simulink model "crearhuerto_Harness11"  (R2020b)
settings: Solver=VariableStepAuto  StartTime=0.0  StopTime=10.0  RelTol=1e-3
settings Model: Creator=Jose  LastModifiedBy=Jose

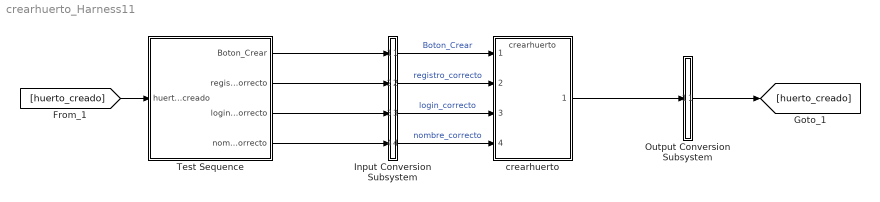
== system crearhuerto_Harness11 ==
  Input Conversion Subsystem : Subsystem  Tag=__SLT_ICS__  Description=|
      | Signal spec.
      | and routing
      settings: AttributesFormatString=%<Description>
  Output Conversion Subsystem : Subsystem  Tag=__SLT_OCS__  Description=|
      | Signal spec.
      | and routing
      settings: AttributesFormatString=%<Description>
  Test Sequence : Test Sequence  TreatAsAtomicUnit=on
  crearhuerto : ModelReference  ModelNameDialog=crearhuerto  SimulationMode=Normal  ModelReferenceVersion=1.12
  wires:
  Test Sequence/1(Boton_Crear) -> Input Conversion Subsystem/1(Inport_1)
  Test Sequence/2(registro_correcto) -> Input Conversion Subsystem/2(Inport_2)
  Test Sequence/3(login_correcto) -> Input Conversion Subsystem/3(Inport_3)
  Test Sequence/4(nombre_correcto) -> Input Conversion Subsystem/4(Inport_4)
  [huerto_creado] -> Test Sequence/1(huerto_creado)
  Output Conversion Subsystem/1(Outport_1) -> [huerto_creado]
  Input Conversion Subsystem/1(Outport_1) -> crearhuerto/1  "Boton_Crear"
  Input Conversion Subsystem/2(Outport_2) -> crearhuerto/2  "registro_correcto"
  Input Conversion Subsystem/3(Outport_3) -> crearhuerto/3  "login_correcto"
  Input Conversion Subsystem/4(Outport_4) -> crearhuerto/4  "nombre_correcto"
  crearhuerto/1 -> Output Conversion Subsystem/1(Inport_1)

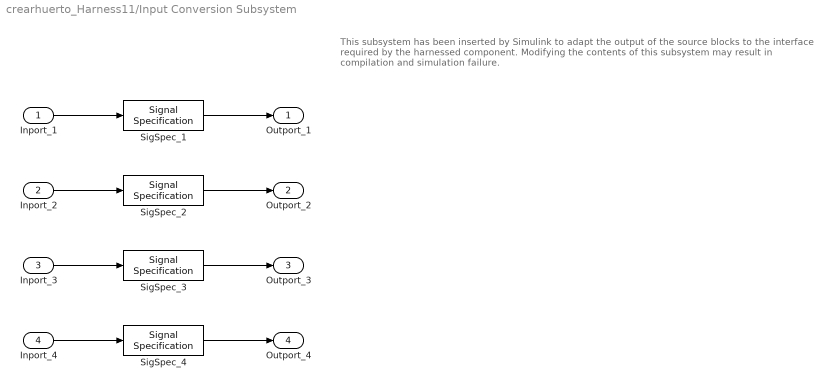
== system crearhuerto_Harness11/Input Conversion Subsystem ==
  note: This subsystem has been inserted by Simulink to adapt the output of the source blocks to the interface required by the harnessed component.
      |  Modifying the contents of this subsystem may result in compilation and simulation failure.
  Inport_1 : Inport
  Inport_2 : Inport  Port=2
  Inport_3 : Inport  Port=3
  Inport_4 : Inport  Port=4
  SigSpec_{1..4} (4 alike) : SignalSpecification  OutDataTypeStr=boolean  Dimensions=[1]  SampleTime=[-1, 0]
  Outport_1 : Outport
  Outport_2 : Outport  Port=2
  Outport_3 : Outport  Port=3
  Outport_4 : Outport  Port=4
  wires:
  SigSpec_1/1 -> Outport_1/1
  Inport_1/1 -> SigSpec_1/1
  SigSpec_2/1 -> Outport_2/1
  Inport_2/1 -> SigSpec_2/1
  SigSpec_3/1 -> Outport_3/1
  Inport_3/1 -> SigSpec_3/1
  SigSpec_4/1 -> Outport_4/1
  Inport_4/1 -> SigSpec_4/1

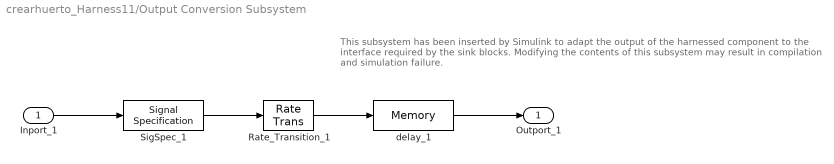
== system crearhuerto_Harness11/Output Conversion Subsystem ==
  note: This subsystem has been inserted by Simulink to adapt the output of the harnessed component to the interface required by the sink blocks.
      |  Modifying the contents of this subsystem may result in compilation and simulation failure.
  Inport_1 : Inport
  Rate_Transition_1 : RateTransition  OutPortSampleTimeOpt=Inherit
  SigSpec_1 : SignalSpecification  OutDataTypeStr=boolean  Dimensions=[1]
  delay_1 : Memory
  Outport_1 : Outport
  wires:
  Inport_1/1 -> SigSpec_1/1
  SigSpec_1/1 -> Rate_Transition_1/1
  Rate_Transition_1/1 -> delay_1/1
  delay_1/1 -> Outport_1/1

== stateflow chart crearhuerto_Harness11/Test Sequence ==
  settings: stateMachineType=SIMPLIFIED_MACHINE
  state Run
    %% Initialize data outputs.
    Boton_Crear = false;
    registro_correcto = false;
    login_correcto = false;
    nombre_correcto = false;
  (default) -> Run
  data: huerto_creado input boolean size=[1]; Boton_Crear output boolean size=[1]; registro_correcto output boolean size=[1]; login_correcto output boolean size=[1]; nombre_correcto output boolean size=[1]
